simulink model "Dyn_PointMass_R2015B"  (R2015b)
settings: Solver=ode4  SolverMode=SingleTasking  StartTime=0.0  StopTime=simInit.TSIM  FixedStep=simInit.dt  MaxStep=simInit.dt  RelTol=1e-3
InitFcn:
  | close all
undefined symbols (not defined in the file): base_windspeed, constr, DE2019, DiscIntNeverNeededParam, ENVMT, Lbooth, loiterStates, params, simInit, T, winchParameter
libraries: simulink x40, simulink_extras x3, dspsigops x1
(part 3 of 5)

== system Dyn_PointMass_R2015B/AirborneSystem/FlightControlSystem/PathFollowingController_SS_2/FlightOnFlatEarth (Retraction&Loitering)/CalculateAttitudeCmds/FlightPathLoopRetraction_Aerodynamic/FlightPathLoopRetraction ==
  F_t_kite : Inport
  F_t_set : Inport  Port=2
  nu_a_path : Inport  Port=3
  flightMode : Inport  Port=4
  sub_flightMode : Inport  Port=5
  StateEstimation_Bus : Inport  Port=6
  Bus Selector : BusSelector  OutputSignals=pos_G_O_m,pathangles_a,airdata,mu_a
  Chart : Stateflow chart  TreatAsAtomicUnit=on
  Compare To Constant1 : simulink/Logic and Bit Operations/Compare To Constant  relop===  const=7  OutDataTypeStr=boolean
  Compare To Constant2 : simulink/Logic and Bit Operations/Compare To Constant  relop===  const=6  OutDataTypeStr=boolean
  Delay : Delay  DelayLength=1  InitialConditionSource=Input port
      settings: InputPortMap=u0,p4
  Delay1 : Delay  DelayLength=1  InitialConditionSource=Input port
      settings: InputPortMap=u0,p4
  Demux : Demux  Outputs=2
  Demux1 : Demux  Outputs=2
  Logical Operator : Logic  Operator=OR  AllPortsSameDT=off  OutDataTypeStr=boolean
  MATLAB Function : MATLAB Function  TreatAsAtomicUnit=on
  Scope : Scope  NumInputPorts=3
  Scope1 : Scope
  Switch : Switch  Criteria=u2 > Threshold
  Transfer Fcn : TransferFcn  Commented=through  Numerator=[10]  Denominator=[1 10]
  inversionPathDynamics : MATLAB Function  TreatAsAtomicUnit=on
  mu_a_c : Outport  PortDimensions=1
  alpha_a_c : Outport  Port=2  PortDimensions=1
  chi_dot_real : Outport  Port=3  PortDimensions=1
  gamma_dot_real : Outport  Port=4  PortDimensions=1
  wires:
  Bus Selector/1 -> inversionPathDynamics/6(pos_O)  "<pos_G_O_m>"
  Demux1/2 -> inversionPathDynamics/8(gamma_a)
  Bus Selector/2 -> Demux1/1  "<pathangles_a>"
  Bus Selector/3 -> inversionPathDynamics/9(airdata), MATLAB Function/1(airdata)  "<airdata>"
  StateEstimation_Bus/1 -> Bus Selector/1
  MATLAB Function/1(L_rq) -> Delay/2
  inversionPathDynamics/1(mu_a_c) -> Delay1/1, mu_a_c/1
  Delay1/1 -> inversionPathDynamics/1(mu_a_c_old)
  Delay/1 -> inversionPathDynamics/11(Lrq_old)
  flightMode/1 -> inversionPathDynamics/3(flightMode)
  nu_a_path/1 -> Demux/1
  Demux/2 -> inversionPathDynamics/5(nu_gamma_a)
  Demux/1 -> inversionPathDynamics/4(nu_chi_a)
  inversionPathDynamics/2(alpha_a_c) -> alpha_a_c/1
  Demux1/1 -> inversionPathDynamics/7(chi_a)
  Bus Selector/4 -> inversionPathDynamics/10(mu_a), Delay1/2  "<mu_a>"
  inversionPathDynamics/5(L_rq) -> Delay/1
  inversionPathDynamics/3(chi_dot_real) -> chi_dot_real/1
  inversionPathDynamics/4(gamma_dot_real) -> gamma_dot_real/1
  F_t_set/1 -> Scope/1, Chart/1(Ftset)
  F_t_kite/1 -> Switch/1, Chart/2(Ftm)
  Chart/1(fset) -> Switch/3, Scope/2
  Switch/1 -> Scope/3, inversionPathDynamics/2(f_t)
  sub_flightMode/1 -> Scope1/1, Chart/3(sub_flightMode), Compare To Constant1/1, Compare To Constant2/1
  Compare To Constant2/1 -> Logical Operator/2
  Compare To Constant1/1 -> Logical Operator/1
  Logical Operator/1 -> Switch/2

== system Dyn_PointMass_R2015B/AirborneSystem/FlightControlSystem/PathFollowingController_SS_2/FlightOnFlatEarth (Retraction&Loitering)/CalculateAttitudeCmds/FlightPathLoopRetraction_Aerodynamic/FlightpathReferenceModels ==
  chi_cmd : Inport
  gamma_cmd : Inport  Port=2
  gamma_hedge : Inport  Port=3
  chi_hedge : Inport  Port=4
  Mux2 : Mux  Inputs=2
  Mux3 : Mux  Inputs=2
  SecondOrderReferenceModel_course : Subsystem  mask{omega0_max=params.w0_chi_retraction_max, zeta0=1, y_max=inf, y_min=-inf, yd_max=inf, yd_min=-inf, y2d_max=inf, y2d_min=-inf}
  SecondOrderReferenceModel_pathangle : Subsystem  mask{omega0_max=params.w0_gamma_retraction_max, zeta0=1, y_max=inf, y_min=-inf, yd_max=inf, yd_min=-inf, y2d_max=inf, y2d_min=-inf}
  xD_ref : Outport
  x_ref : Outport  Port=2
  wires:
  gamma_hedge/1 -> SecondOrderReferenceModel_pathangle/2(hedge)
  chi_hedge/1 -> SecondOrderReferenceModel_course/2(hedge)
  gamma_cmd/1 -> SecondOrderReferenceModel_pathangle/1(y_cmd)
  chi_cmd/1 -> SecondOrderReferenceModel_course/1(y_cmd)
  Mux3/1 -> xD_ref/1
  Mux2/1 -> x_ref/1
  SecondOrderReferenceModel_course/1(y_ref) -> Mux2/1
  SecondOrderReferenceModel_pathangle/1(y_ref) -> Mux2/2
  SecondOrderReferenceModel_course/2(y_ref_dot) -> Mux3/1
  SecondOrderReferenceModel_pathangle/2(y_ref_dot) -> Mux3/2

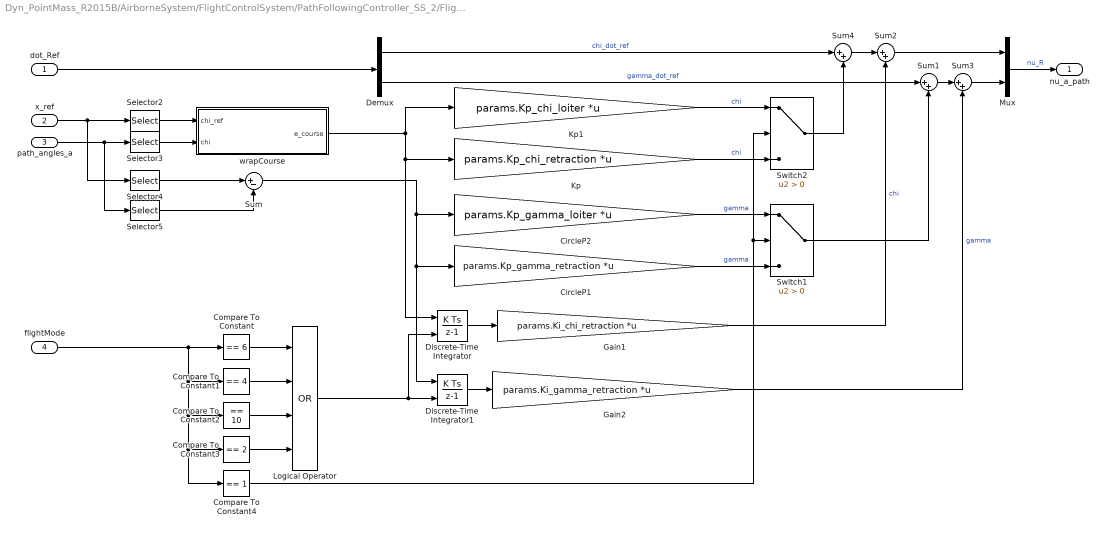
== system Dyn_PointMass_R2015B/AirborneSystem/FlightControlSystem/PathFollowingController_SS_2/FlightOnFlatEarth (Retraction&Loitering)/CalculateAttitudeCmds/FlightPathLoopRetraction_Aerodynamic/PIController_opt ==
  dot_Ref : Inport
  x_ref : Inport  Port=2
  path_angles_a : Inport  Port=3
  flightMode : Inport  Port=4
  CircleP1 : Gain  Gain=params.Kp_gamma_retraction  Multiplication=Matrix(K*u)
  CircleP2 : Gain  Gain=params.Kp_gamma_loiter  Multiplication=Matrix(K*u)
  Compare To Constant : simulink/Logic and Bit Operations/Compare To Constant  relop===  const=6  OutDataTypeStr=boolean
  Compare To Constant1 : simulink/Logic and Bit Operations/Compare To Constant  relop===  const=4  OutDataTypeStr=boolean
  Compare To Constant2 : simulink/Logic and Bit Operations/Compare To Constant  relop===  const=10  OutDataTypeStr=boolean
  Compare To Constant3 : simulink/Logic and Bit Operations/Compare To Constant  relop===  const=2  OutDataTypeStr=boolean
  Compare To Constant4 : simulink/Logic and Bit Operations/Compare To Constant  relop===  const=1  OutDataTypeStr=boolean
  Demux : Demux  Outputs=2
  Discrete-Time Integrator : DiscreteIntegrator  ExternalReset=either  InitialConditionSetting=State (most efficient)  SampleTime=-1  ICPrevOutput=DiscIntNeverNeededParam  ICPrevScaledInput=DiscIntNeverNeededParam
  Discrete-Time Integrator1 : DiscreteIntegrator  ExternalReset=either  InitialConditionSetting=State (most efficient)  SampleTime=-1  ICPrevOutput=DiscIntNeverNeededParam  ICPrevScaledInput=DiscIntNeverNeededParam
  Gain1 : Gain  Gain=params.Ki_chi_retraction  Multiplication=Matrix(K*u) (u vector)
  Gain2 : Gain  Gain=params.Ki_gamma_retraction  Multiplication=Matrix(K*u) (u vector)
  Kp : Gain  Gain=params.Kp_chi_retraction  Multiplication=Matrix(K*u)
  Kp1 : Gain  Gain=params.Kp_chi_loiter  Multiplication=Matrix(K*u)
  Logical Operator : Logic  Operator=OR  Inputs=4  AllPortsSameDT=off  OutDataTypeStr=boolean
  Mux : Mux  Inputs=2
  Selector2 : Selector  InputPortWidth=2  IndexOptions=Index vector (dialog)  Indices=1  OutputSizes=1
  Selector3 : Selector  InputPortWidth=2  IndexOptions=Index vector (dialog)  Indices=1  OutputSizes=1
  Selector4 : Selector  InputPortWidth=2  IndexOptions=Index vector (dialog)  Indices=2  OutputSizes=1
  Selector5 : Selector  InputPortWidth=2  IndexOptions=Index vector (dialog)  Indices=2  OutputSizes=1
  Sum : Sum  Inputs=|+-
  Sum{1..4} (4 alike) : Sum  Inputs=|++
  Switch1 : Switch  Criteria=u2 > Threshold
  Switch2 : Switch  Criteria=u2 > Threshold
  wrapCourse : MATLAB Function  TreatAsAtomicUnit=on
  nu_a_path : Outport
  wires:
  Compare To Constant3/1 -> Logical Operator/4
  Logical Operator/1 -> Discrete-Time Integrator/2, Discrete-Time Integrator1/2
  flightMode/1 -> Compare To Constant2/1, Compare To Constant4/1, Compare To Constant3/1, Compare To Constant1/1, Compare To Constant/1
  Mux/1 -> nu_a_path/1  "nu_R"
  dot_Ref/1 -> Demux/1
  Demux/1 -> Sum4/1  "chi_dot_ref"
  Kp/1 -> Switch2/3  "chi"
  Sum4/1 -> Sum2/1
  wrapCourse/1(e_course) -> Kp/1, Discrete-Time Integrator/1, Kp1/1
  Demux/2 -> Sum1/1  "gamma_dot_ref"
  CircleP1/1 -> Switch1/3  "gamma"
  Sum1/1 -> Sum3/1
  Sum/1 -> Discrete-Time Integrator1/1, CircleP1/1, CircleP2/1
  Compare To Constant/1 -> Logical Operator/1
  Compare To Constant1/1 -> Logical Operator/2
  Compare To Constant2/1 -> Logical Operator/3
  Discrete-Time Integrator1/1 -> Gain2/1
  path_angles_a/1 -> Selector5/1, Selector3/1
  Selector4/1 -> Sum/1
  Selector2/1 -> wrapCourse/1(chi_ref)
  x_ref/1 -> Selector4/1, Selector2/1
  Gain1/1 -> Sum2/2  "chi"
  Gain2/1 -> Sum3/2  "gamma"
  Discrete-Time Integrator/1 -> Gain1/1
  Sum2/1 -> Mux/1
  Sum3/1 -> Mux/2
  Selector5/1 -> Sum/2
  Selector3/1 -> wrapCourse/2(chi)
  Compare To Constant4/1 -> Switch2/2, Switch1/2
  Switch2/1 -> Sum4/2
  Kp1/1 -> Switch2/1  "chi"
  CircleP2/1 -> Switch1/1  "gamma"
  Switch1/1 -> Sum1/2

== system Dyn_PointMass_R2015B/AirborneSystem/FlightControlSystem/PathFollowingController_SS_2/FlightOnFlatEarth (Retraction&Loitering)/GuidanceFlatEarth/LoiteringGuidance/Subsystem ==
  v_k_O : Inport
  h_cmd : Inport  Port=2
  h : Inport  Port=3
  Asin : Trigonometry  Operator=asin
  Divide : Product  Inputs=*/
  Dot Product : DotProduct  InputSameDT=on  OutDataTypeStr=Inherit: Inherit via internal rule
  Gain2 : Gain  Gain=-1
  Gain3 : Gain  Gain=loiterStates.kp_h
  Saturation : Saturate  UpperLimit=50*pi/180  LowerLimit=-50*pi/180
  Saturation1 : Saturate  UpperLimit=1  LowerLimit=-1
  Selector : Selector  InputPortWidth=3  IndexOptions=Index vector (dialog)  Indices=3  OutputSizes=1
  Sqrt : Sqrt  SaturateOnIntegerOverflow=on
  Sum2 : Sum  Inputs=|-+
  gamma_k_cmd : Outport
  wires:
  h_cmd/1 -> Sum2/2
  Saturation/1 -> gamma_k_cmd/1
  Selector/1 -> Gain2/1
  Gain2/1 -> Sum2/1
  Sum2/1 -> Gain3/1
  Sqrt/1 -> Divide/2
  Divide/1 -> Saturation1/1
  Dot Product/1 -> Sqrt/1
  v_k_O/1 -> Dot Product/1, Dot Product/2
  h/1 -> Selector/1
  Asin/1 -> Saturation/1
  Saturation1/1 -> Asin/1
  Gain3/1 -> Divide/1

== system Dyn_PointMass_R2015B/AirborneSystem/FlightControlSystem/PathFollowingController_SS_2/FlightOnFlatEarth (Retraction&Loitering)/GuidanceFlatEarth/Retraction_Nav/Subsystem ==
  In1 : Inport
  Dot Product3 : DotProduct  InputSameDT=on  OutDataTypeStr=Inherit: Inherit via internal rule
  Sqrt1 : Sqrt  SaturateOnIntegerOverflow=on
  Out1 : Outport
  wires:
  In1/1 -> Dot Product3/1, Dot Product3/2
  Sqrt1/1 -> Out1/1
  Dot Product3/1 -> Sqrt1/1

== system Dyn_PointMass_R2015B/AirborneSystem/FlightControlSystem/PathFollowingController_SS_2/FlightOnFlatEarth (Retraction&Loitering)/GuidanceFlatEarth/Retraction_Nav/hold1 ==
  In1 : Inport
  Delay2 : Delay  DelayLength=1  InitialConditionSource=Input port  InitialCondition=zeros(3,1)
      settings: InputPortMap=u0,p4
  Out1 : Outport
  wires:
  In1/1 -> Delay2/2
  Delay2/1 -> Out1/1, Delay2/1

== system Dyn_PointMass_R2015B/AirborneSystem/FlightControlSystem/PathFollowingController_SS_2/FlightOnFlatEarth (Retraction&Loitering)/CalculateAttitudeCmds/FlightPathLoopRetraction_Aerodynamic/FlightpathReferenceModels/SecondOrderReferenceModel_course ==
  y_cmd : Inport
  hedge : Inport  Port=2
  Constant : Constant  Value=omega0_max
  Discrete-Time Integrator : DiscreteIntegrator  InitialConditionSetting=State (most efficient)  SampleTime=-1  LimitOutput=on  UpperSaturationLimit=y_max  LowerSaturationLimit=y_min  ICPrevOutput=DiscIntNeverNeededParam  ICPrevScaledInput=DiscIntNeverNeededParam
  Discrete-Time Integrator1 : DiscreteIntegrator  InitialConditionSetting=State (most efficient)  SampleTime=-1  LimitOutput=on  UpperSaturationLimit=yd_max  LowerSaturationLimit=yd_min  ICPrevOutput=DiscIntNeverNeededParam  ICPrevScaledInput=DiscIntNeverNeededParam
  Gain2 : Gain  Gain=2*zeta0
  Product : Product  Inputs=3
  Product1 : Product
  Saturation : Saturate  UpperLimit=y_max  LowerLimit=y_min
  Saturation1 : Saturate  UpperLimit=y2d_max  LowerLimit=y2d_min
  Sum : Sum  Inputs=|+-
  Sum2 : Sum  Inputs=|+-
  calcualteCourseErrorAndWrap : MATLAB Function  TreatAsAtomicUnit=on
  wrapto2pi : MATLAB Function  TreatAsAtomicUnit=on
  y_ref : Outport
  y_ref_dot : Outport  Port=2
  wires:
  Product1/1 -> Gain2/1
  Constant/1 -> Product1/2, Product/3, Product/1
  Discrete-Time Integrator/1 -> wrapto2pi/1(u)
  Product/1 -> Sum/1
  y_cmd/1 -> Saturation/1
  Discrete-Time Integrator1/1 -> y_ref_dot/1, Product1/1, Sum2/1  "v:_r"
  Sum/1 -> Saturation1/1
  Gain2/1 -> Sum/2
  calcualteCourseErrorAndWrap/1(e_course) -> Product/2
  Saturation1/1 -> Discrete-Time Integrator1/1  "v_dot_r"
  Saturation/1 -> calcualteCourseErrorAndWrap/1(chi_ref)
  Sum2/1 -> Discrete-Time Integrator/1
  hedge/1 -> Sum2/2
  wrapto2pi/1(y) -> calcualteCourseErrorAndWrap/2(chi), y_ref/1

== system Dyn_PointMass_R2015B/AirborneSystem/FlightControlSystem/PathFollowingController_SS_2/FlightOnFlatEarth (Retraction&Loitering)/CalculateAttitudeCmds/FlightPathLoopRetraction_Aerodynamic/FlightpathReferenceModels/SecondOrderReferenceModel_pathangle ==
  y_cmd : Inport
  hedge : Inport  Port=2
  Constant : Constant  Value=omega0_max
  Discrete-Time Integrator : DiscreteIntegrator  InitialConditionSetting=State (most efficient)  SampleTime=-1  LimitOutput=on  UpperSaturationLimit=y_max  LowerSaturationLimit=y_min  ICPrevOutput=DiscIntNeverNeededParam  ICPrevScaledInput=DiscIntNeverNeededParam
  Discrete-Time Integrator1 : DiscreteIntegrator  InitialConditionSetting=State (most efficient)  SampleTime=-1  LimitOutput=on  UpperSaturationLimit=yd_max  LowerSaturationLimit=yd_min  ICPrevOutput=DiscIntNeverNeededParam  ICPrevScaledInput=DiscIntNeverNeededParam
  Gain2 : Gain  Gain=2*zeta0
  Product : Product  Inputs=3
  Product1 : Product
  Saturation : Saturate  UpperLimit=y_max  LowerLimit=y_min
  Saturation1 : Saturate  UpperLimit=y2d_max  LowerLimit=y2d_min
  Sum : Sum  Inputs=|+-
  Sum1 : Sum  Inputs=|+-
  Sum2 : Sum  Inputs=|+-
  y_ref : Outport
  y_ref_dot : Outport  Port=2
  wires:
  Product1/1 -> Gain2/1
  Constant/1 -> Product1/2, Product/3, Product/1
  Product/1 -> Sum/1
  y_cmd/1 -> Saturation/1
  Discrete-Time Integrator1/1 -> y_ref_dot/1, Product1/1, Sum2/1  "v:_r"
  Sum/1 -> Saturation1/1
  Gain2/1 -> Sum/2
  Sum1/1 -> Product/2
  Saturation1/1 -> Discrete-Time Integrator1/1  "v_dot_r"
  Saturation/1 -> Sum1/1
  Sum2/1 -> Discrete-Time Integrator/1
  hedge/1 -> Sum2/2
  Discrete-Time Integrator/1 -> y_ref/1, Sum1/2

== stateflow chart Dyn_PointMass_R2015B/AirborneSystem/FlightControlSystem/PathFollowingController_SS_2/FlightOnFlatEarth (Retraction&Loitering)/CalculateAttitudeCmds/FlightPathLoopRetraction_Aerodynamic/FlightPathLoopRetraction/Chart ==
  settings: updateMethod=DISCRETE  sampleTime=0.1
  state ReducedSetforce
    during: fset = 0 ;
    during: t = t + 1;
  state Setforce
    during: fset = Ftset;
    entry: t=0;
  Setforce -> ReducedSetforce [commented out] : [Ftm>Ftset+1000]
  (default) -> Setforce
  Setforce -> ReducedSetforce : [sub_flightMode==6 || sub_flightMode == 7]
  ReducedSetforce -> Setforce : [sub_flightMode==8]
  ReducedSetforce -> Setforce [commented out] : [Ftm<Ftset-1000]
  data: Ftset input; Ftm input; fset output; t local; sub_flightMode input

== matlab function Dyn_PointMass_R2015B/ParticleTetherModel/Tether_SS_5/Tether_Dynamics ==
  data: kitePos input; tetherPos output size=[3,T.np]; kiteVel input; windVel input; tetherLength input; x input; Ft_Ground output; Ft_Kite output; Fvec output; x output; ENVMT parameter; T parameter
% Copyright 2021 Delft University of Technology
%
% Licensed under the Apache License, Version 2.0 (the "License");
% you may not use this file except in compliance with the License.
% You may obtain a copy of the License at
%
%      http://www.apache.org/licenses/LICENSE-2.0
%
% Unless required by applicable law or agreed to in writing, software
% distributed under the License is distributed on an "AS IS" BASIS,
% WITHOUT WARRANTIES OR CONDITIONS OF ANY KIND, either express or implied.
% See the License for the specific language governing permissions and
% limitations under the License.

function [tetherPos, Ft_Ground, Ft_Kite, Fvec, x]= ...
    Tether_QuasiStatic(kitePos, kiteVel, windVel, tetherLength, x, ENVMT, T)
%#codegen

%Tether_QuasiStatic Trust-region dogleg nonlinear systems of equation
%   solver to determine the tether shape and forces.
%
%   Tether_QuasiStatic is based on the matlab implementation that 
%   solves a system of nonlinear equations using a dogleg
%   trust region approach.  The algorithm implemented is similar in nature
%   to the FORTRAN program HYBRD1 of J.J. More', B.S. Garbow and K.E. 
%   Hillstrom, User Guide for MINPACK 1, Argonne National Laboratory, 
%   Rept. ANL-80-74, 1980, which itself was based on the program CALFUN 
%   of M.J.D. Powell, A Fortran subroutine for solving systems of
%   nonlinear algebraic equations, Chap. 7 in P. Rabinowitz, ed.,
%   Numerical Methods for Nonlinear Algebraic Equations, Gordon and
%   Breach, New York, 1970.
%
%   Addapted by Ir. D. Eijkelhof (TU Delft) from 1990-2019 Matlab version 
%   The MathWorks, Inc.
% NOTE: From Matlab 2020b Matlab's Levenberg–Marquardt algorithm in the
% command "solve" can be directly used in codegen and might be
% faster. Due to availability of only matlab R2019B and lower, an own
% implementation had to be used in order the execute codegen.
%
% Syntax:  [tetherPos, Ft_Ground, Ft_Kite, Fvec, x]= ...
%     Tether_QuasiStatic(kitePos, kiteVel, windVel, tetherLength, x, ENVMT, T)
%
% NOTE: 'x' passed in and returned in column vector form.
%
% Throughout this routine 'x', 'F', 'xvec', 'xTrial', 'Fvec' and 'FTrial' are vectors.
%
% Inputs:
%    tetherPos  - Position vectors of tether particles
%    Ft_Ground  - Tether force magnitude at the ground station
%    Ft_Kite    - Tether force vector at the kite
%    Fvec       - Error between tether end and kite position (3D)
%    x          - Tether ground segment orientation and magnitude
%
% Outputs:
%    kitePos        - Kite position vector in wind reference frame
%    kiteVel        - Kite velocity vector in wind reference frame
%    windVel        - Wind velocity vector in wind reference frame
%    ENVMT          - Environmental parameters
%    tetherLength   - Reeled-out tether length determined by the winch
%    x              - Initial tether ground segment orientation and magnitude
%    T              - Tether dimensions and material properties
%
% Other m-files required: none
%
% Subfunctions: Objfunc    : Calculate difference between tether end and
%                            kite given tether ground segment orientation
%                            and magnitude.
%               testStop   : Test convergence criteria's
%               dogleg_tem : approximately solves trust region subproblem
%                            via a dogleg approach. 
%               lm_FD_J    : Determines the jacobian matrix by forward
%                            differencing
%
% MAT-files required: none
%
% Author: Dylan Eijkelhof, M.Sc.
% Delft University of Technology
% email address: d.eijkelhof@tudelft.nl  
% December 2019; Last revision: 16-March-2021

%------------- BEGIN CODE --------------
    
    [Fvec,T0,pj,~] = Objfunc(x,kitePos,kiteVel,windVel,tetherLength,ENVMT,T);
    
    xvec = x(:);         % vector representation of x
    % Convert values to full to avoid unnecessary sparse operation overhead
    % Initial x
    Fvec = full(Fvec); 
    
    % Set tolerances
    maxfunc     = 100*5;
    maxit       = 1000;
    tolf        = 1e-9;
    tolfunvalue = 1e-6;
    tolx        = 1e-6;
    tolobj      = 1e-6;
    
    nVar        = 3; % for codegen it worked better than numel(x)

    % Initialize local arrays.
    d           = zeros(nVar,1);

    % Initialize other trust region parameters.
    Delta       = 1e0;
    DeltaMax    = 1e10;
    eta1        = T.eta1;
    eta2        = T.eta2;
    alpha1      = T.alpha1;
    alpha2      = T.alpha2;

    % Extra initializations.
    iter        = 0;
    numFevals   = 1;

    stepAccept  = true;
    normd       = 0.0e0;
    objold      = 1.0e0;
    obj         = 0.5*(Fvec'*Fvec);  % Initial Fvec computed above

    numFDfevals = 0; %#ok<NASGU>
    JAC         = zeros(3,3); %#ok<PREALL> % pre-allocate derivative array

    %%%%%%%%%%%%%%%%%%%%%%% Calculate Jacobian at x0 %%%%%%%%%%%%%%%%%%
    [JAC,numFDfevals] = lm_FD_J(x, 0.1*ones(3,1),kitePos, kiteVel, ...
        windVel, tetherLength, ENVMT, T);

    % Increment the number of function evaluations with those used in the
    % finite difference calls.
    numFevals = numFevals + numFDfevals;

    grad = JAC'*Fvec;
    normgradinf = norm(grad,inf);

    % Test convergence at initial point.
    [done,~] = testStop(normgradinf,tolf,tolfunvalue,tolx,...
         stepAccept,iter,maxit,numFevals,maxfunc,Delta,normd,...
         obj,objold,d,xvec,tolobj,Fvec);

    % Beginning of main iteration loop.
    while ~done
    	iter = iter + 1;

    	% Compute step, d, using dogleg approach.
    	[d,quadObj,normd,normdscal] = ...
           dogleg(nVar,Fvec,JAC,grad,Delta);

        % Compute the model reduction given by d (pred).
        pred = -quadObj;

        % Compute the trial point, xTrial. Limit to positive value
        xTrial = xvec + d;
        if xTrial(3) < 0
            xTrial(3) = 1e-3;
        end

        % Evaluate nonlinear equations and objective at trial point.
        [F,T0,pj,~] = Objfunc(xTrial,kitePos,kiteVel,windVel,tetherLength,...
            ENVMT,T);
      
      
        numFevals = numFevals + 1;
        FTrial    = full(F(:)); % make FTrial a vector, convert to full
        objTrial  = 0.5*(FTrial'*FTrial); 

        % Compute the actual reduction given by xTrial (ared).
        ared      = obj - objTrial;

        % Compute ratio = ared/pred.
        if pred <= 0 % reject step
            ratio = 0;
        else
            ratio = ared/pred;
        end

        currTrialWellDefined = isfinite(objTrial);

        if ratio > eta1 && currTrialWellDefined % accept step.

            xvec    = xTrial; 
            objold  = obj; 
            obj     = objTrial;
            x(:)    = xvec; % update matrix representation
        
            %%%%%%%%%%%%%%%%%%%%%% Calculate New Jacobian %%%%%%%%%%%%%%%%%
            if iter == 1 || mod(iter,2*size(x,1))==0
                [JAC,numFDfevals] = lm_FD_J(x, 0.01*ones(3,1),kitePos, kiteVel, windVel, tetherLength, ENVMT, T);

                numFevals = numFevals + numFDfevals;
            else
                JAC = JAC + ((FTrial-Fvec-JAC*d)*d')/(d'*d);
            end
        
            Fvec        = FTrial; 
            grad        = JAC'*Fvec;
            normgradinf = norm(grad,inf);

            stepAccept  = true;
        else % reject step.
            stepAccept  = false;
        end 


        % Update trust region radius.
        if ~currTrialWellDefined
            % Shrink the trust region if any element of the function vector
            % at the new step is not defined (i.e. it's inf/NaN/complex). The
            % update for Delta in this case follows that in snls.
            Delta = min(normdscal/20,Delta/20);
        elseif ratio < eta1
            Delta = alpha2*normdscal;
        elseif ratio >= eta2
            Delta = max(Delta,alpha1*normdscal);
        end
        Delta = min(Delta,DeltaMax);

        % Check for termination.
        [done,~] = testStop(normgradinf,tolf,tolfunvalue,tolx,...
            stepAccept,iter,maxit,numFevals,maxfunc,Delta,normd,...
            obj,objold,d,xvec,tolobj,Fvec);
    end

    % Optimization is finished.  
    Ft_Ground   = x(3);
    Ft_Kite     = T0;
    tetherPos   = pj;
end

%%%%%%%%%%%%%%%%%%%%%%%%%%%%%%%%%%%%%%%%%%%%%%%%%%%%%%%%%%%%%%%
function [Fobj,T0,pj,p0] = Objfunc(stateVec,kitePos, kiteVel, windVel,...
                              tetherLength, ENVMT, T)
    Ns = size(windVel,2);       % number of masses
    Ls = tetherLength/(Ns+1);   % segment length
    mj = T.rho_t * Ls;          % segment mass

    p = kitePos;                % input aircraft position
    v = kiteVel;                % input aircraft velocity

    theta = stateVec(1);
    phi = stateVec(2);
    Tn = stateVec(3);

    omega_t = cross(p./(norm(p)^2),v);

    E = T.E;
    A = T.A;

    FT = zeros(3,Ns); % Tension forces
    Fd = zeros(3,Ns); % Drag forces
    pj = zeros(3,Ns); % Mass positions
    vj = zeros(3,Ns); % Mass velocities
    aj = zeros(3,Ns); % Mass accellerations

    % First element from ground station (Ns)
    FT(:,Ns) = Tn.*[sin(theta)* cos(phi); sin(phi); cos(theta)*cos(phi)];
    pj(:,Ns) = Ls.*[sin(theta)* cos(phi); sin(phi); cos(theta)*cos(phi)];
    vj(:,Ns) = dot(v,p./norm(p)) .* (p./norm(p)) + cross(omega_t,pj(:,Ns));
    aj(:,Ns) = cross(omega_t,cross(omega_t,pj(:,Ns)));
    
    % Drag calculation first element
    v_a_p = vj(:,Ns) - windVel(:,Ns);
    if all(abs(v_a_p)<1e-3)
        Fd(:,Ns) = [0;0;0];
    else
        v_a_p_t = dot((pj(:,Ns))/norm(pj(:,Ns)),v_a_p)*...
            ((pj(:,Ns))/norm(pj(:,Ns)));
        v_a_p_n = v_a_p - v_a_p_t;
        Fd(:,Ns) = -0.5 * ENVMT.rhos * Ls * T.d_tether * T.CD_tether * ...
            norm(v_a_p_n) * v_a_p_n; % particle drag
    end
    
    % All other segments and masses except for segment connected to the kite
    for i = Ns:-1:2
        if i == Ns
            FT(:,i-1) = (mj+0.5*mj).*aj(:,i) + FT(:,i) - Fd(:,i) + ...
                [0;0;(mj+0.5*mj)*ENVMT.g];
        else
            FT(:,i-1) = mj.*aj(:,i) + FT(:,i) - Fd(:,i) + [0;0;mj*ENVMT.g];
        end

        l_i_1 = (norm(FT(:,i-1))/(E*A) + 1)*Ls;
        
        pj(:,i-1) = pj(:,i) + l_i_1.*(FT(:,i-1)/norm(FT(:,i-1)));       
        vj(:,i-1) = dot(v,p./norm(p)) .* (p./norm(p)) + cross(omega_t,pj(:,i-1));
        aj(:,i-1) = cross(omega_t,cross(omega_t,pj(:,i-1)));
        
        % Drag calculation
        v_a_p = vj(:,i) - windVel(:,i);
        if all(abs(v_a_p)<1e-3)
            Fd(:,i-1) = [0;0;0];
        else
            v_a_p_t = dot((pj(:,i-1)-pj(:,i))/norm(pj(:,i-1)-pj(:,i)),v_a_p) * ...
                ((pj(:,i-1)-pj(:,i))/norm(pj(:,i-1)-pj(:,i)));
            v_a_p_n = v_a_p - v_a_p_t;
            Fd(:,i-1) = -0.5 * ENVMT.rhos * Ls * T.d_tether * T.CD_tether * ...
                norm(v_a_p_n) * v_a_p_n; % particle drag
        end
    end
    
    T0 = (mj+0.5*mj).*aj(:,1) + FT(:,1) - Fd(:,1) + [0;0;(mj+0.5*mj)*ENVMT.g];
    l_i_1 = (norm(T0)/(E*A) + 1)*Ls;
    p0 = pj(:,1) + l_i_1.*(T0/norm(T0));
    
    Fobj = p-p0;
end
%%%%%%%%%%%%%%%%%%%%%%%%%%%%%%%%%%%%%%%%%%%%%%%%%%%%%%%%%%%%%%%
function [done,EXITFLAG] = testStop(normgradinf,tolf,tolfunvalue,...
        tolx,stepAccept,iter,maxit,numFevals,maxfunc,Delta,normd,...
        obj,objold,d,xvec,tolobj,Fvec)
    %testStop checks the termination criteria for TRUSTNLEQN.

    done = false;
    EXITFLAG = 0;

    % Check termination criteria.

    if stepAccept && normgradinf < tolf
      EXITFLAG = 1;
      done = true;
      
    elseif iter > 1 && max(abs(d)./(abs(xvec)+1)) < max(tolx^2,eps)
       EXITFLAG = 2;
       done = true;
       
    elseif iter > 1 && stepAccept && normd < 0.9*Delta ...
                    && abs(objold-obj) < max(tolfunvalue^2,eps)*(1+abs(objold))
      EXITFLAG = 3;
      done = true;
      
    elseif iter > 1 && norm(Fvec) < tolobj
      EXITFLAG = 4;
      done = true;
      
    elseif Delta < 2*eps
      EXITFLAG = -3;
      done = true;
      
    elseif iter >= maxit
      EXITFLAG = 0;
      done = true;
      
    elseif numFevals >= maxfunc
      EXITFLAG = 0;
      done = true;
    end  
end
%%%%%%%%%%%%%%%%%%%%%%%%%%%%%%%%%%%%%%%%%%%%%%%%%%%%%%%%%%%%%%%
function [step,quadObj,normStep,normStepScal] = ...
    dogleg(nvar,F,JAC,grad,Delta)
%dogleg approximately solves trust region subproblem via a dogleg approach.
%
%   dogleg finds an approximate solution d to the problem:
%
%     min_d      f + g'd + 0.5*d'Bd
%
%     subject to ||Dd|| <= Delta
%
%   where g is the gradient of f, B is a Hessian approximation of f, D is a
%   diagonal scaling matrix and Delta is a given trust region radius.

%   Copyright 1990-2012 The MathWorks, Inc.
%   $Revision: 1.1.6.7 $  $Date: 2012/08/21 01:08:20 $

% NOTE: The scaling matrix D above is called scalMat in this routine.

% Compute scaled gradient and other scaled terms.
grad2 = grad;
normgradscal = norm(grad);

if normgradscal >= eps
    % First compute the Cauchy step (in scaled space).
    dCauchy = -(Delta/normgradscal)*grad;
    JACvec = JAC*grad2;
    denom = Delta*(JACvec'*JACvec);
    tauterm = normgradscal^3/denom;
    tauC = min(1,tauterm);
    dCauchy = tauC*dCauchy;
    
    % Compute quadratic objective at Cauchy point.
    JACvec = JAC*(dCauchy); 
    objCauchy = grad'*dCauchy + 0.5*(JACvec'*JACvec);   
    normdCauchy = min(norm(dCauchy),Delta);
else
    % Set Cauchy step to zero step and continue.
    objCauchy = 0;
    normdCauchy = 0;
    dCauchy = zeros(nvar,1);
end

if Delta - normdCauchy < eps
    % Take the Cauchy step if it is at the boundary of the trust region.
    step = dCauchy; quadObj = objCauchy;
else
    % Compute the Gauss-Newton step (in scaled space).
    
    dNewton = -JAC\F;
    
    if any(~isfinite(dNewton))
        % Take the Cauchy step if the Gauss-Newton step gives bad values.
        step = dCauchy; quadObj = objCauchy;
    else 
        normdNewt = norm(dNewton);
        if normdNewt <= Delta
            % Use the Newton direction as the trial step
            step = dNewton;
        else
            % Find the intersect point along dogleg path.
            Delta2 = Delta^2;
            normdCauchy2 = min(normdCauchy^2,Delta2);
            normdNewt2 = normdNewt^2;
            dCdN = dCauchy'*dNewton;
            dCdNdist2 = max((normdCauchy2+normdNewt2-2*dCdN),0);
            
            if dCdNdist2 == 0
                Lambda = 0;
            else
                % Stable method for solving 1-D quadratic
                a = 0.5*dCdNdist2;
                b = dCdN - normdCauchy2;
                c = 0.5*(normdCauchy2 - Delta2);
                q = -0.5*(b + sign(b)*sqrt(b^2 - 4*a*c));
                if b > 0
                    Lambda = c/q; 
                else
                    Lambda = q/a;
                end

                % Make sure we take a finite step,
                % (check for poorly scaled/infinite directions).
                if ~isfinite(Lambda)
                    Lambda = 0; % Take Cauchy step
                end
            end
            step = dCauchy + Lambda*(dNewton-dCauchy);
        end
        % Compute quadratic objective at trial point.
        JACvec = JAC*(step);
        quadObj = grad'*step + 0.5*(JACvec'*JACvec);
        
        % Compare Cauchy step and trial step (Newton or intersection)
        if objCauchy < quadObj
            step = dCauchy; quadObj = objCauchy;
        end
    end
end

% The step computed was the scaled step.  Unscale it.
normStepScal = norm(step);
normStep = norm(step);
end
 %%%%%%%%%%%%%%%%%%%%%%%%%%%%%%%%%%%%%%%%%%%%%%%%%%%%%%%%%%%%%%%
function [J,numFDfevals] = lm_FD_J(x, dp,kitePos, kiteVel, windVel, ...
                                tetherLength, ENVMT, T)

 m      = 3;                         % number of data points
 n      = 3;                         % number of parameters

 ps     = x; 
 J      = zeros(m,n); 
 del    = zeros(n,1);                % initialize Jacobian to Zero
 
 for j=1:n                           % START --- loop over all parameters

   del(j) = dp(j) * (1+abs(x(j)));   % parameter perturbation
   x(j)   = ps(j) + del(j);          % perturb parameter x(j)

   if del(j) ~= 0
     [y1,~,~,~] = Objfunc(x,kitePos, kiteVel, windVel, ...
         tetherLength, ENVMT, T);
     
     x(j) = ps(j) - del(j);
     [y,~,~,~] = Objfunc(x,kitePos, kiteVel, windVel, ...
         tetherLength, ENVMT, T);
     
     J(:,j) = (y1-y) ./ (2 .* del(j));
   end

   x(j) = ps(j);                     % restore x(j)

 end
 numFDfevals = 2;
                                     % END --- loop over all parameters
end

== matlab function Dyn_PointMass_R2015B/AirborneSystem/FlightControlSystem/PathFollowingController_SS_2/FlightOnFlatEarth (Retraction&Loitering)/CalculateAttitudeCmds/FlightPathLoopRetraction_Aerodynamic/FlightPathLoopRetraction/MATLAB Function ==
  data: L_rq output; airdata input; DE2019 parameter; constr parameter; ENVMT parameter
% Copyright 2021 Delft University of Technology
%
% Licensed under the Apache License, Version 2.0 (the "License");
% you may not use this file except in compliance with the License.
% You may obtain a copy of the License at
%
%      http://www.apache.org/licenses/LICENSE-2.0
%
% Unless required by applicable law or agreed to in writing, software
% distributed under the License is distributed on an "AS IS" BASIS,
% WITHOUT WARRANTIES OR CONDITIONS OF ANY KIND, either express or implied.
% See the License for the specific language governing permissions and
% limitations under the License.

function L_rq = fcn(airdata, DE2019,constr, ENVMT)
%fcn - Calculate required lift force
%
% Inputs:
%    airdata     - Airspeed, aoa, sideslip angle
%    DE2019     - Aircraft characteristics
%    constr     - Constraint, maximum lift
%
% Outputs:
%    L_rq    - Required lift
%
% Author: Sebastian Rapp, Ph.D., Revised by: Dylan Eijkelhof, M.Sc.
% Delft University of Technology
% email address: s.rapp@tudelft.nl
% email address: d.eijkelhof@tudelft.nl
% December 2019; Last revision: 06-October-2020

%-------------	BEGIN CODE	--------------

L_rq =  min( 0.5*ENVMT.rhos*DE2019.S_wing*airdata(1)^2 * (DE2019.CL0+DE2019.CL_alpha*airdata(2) ),constr.F_T_max); % max. negative lift

%-------------	 END CODE	--------------
end

== matlab function Dyn_PointMass_R2015B/AirborneSystem/FlightControlSystem/PathFollowingController_SS_2/FlightOnFlatEarth (Retraction&Loitering)/CalculateAttitudeCmds/FlightPathLoopRetraction_Aerodynamic/FlightPathLoopRetraction/inversionPathDynamics ==
  data: mu_a_c_old input; f_t input; flightMode input; nu_chi_a input; mu_a_c output; nu_gamma_a input; DE2019 parameter; pos_O input; chi_a input; gamma_a input; airdata input; mu_a input; constr parameter; alpha_a_c output; chi_dot_real output; gamma_dot_real output; ENVMT parameter; L_rq output; Lrq_old input
% Copyright 2021 Delft University of Technology
%
% Licensed under the Apache License, Version 2.0 (the "License");
% you may not use this file except in compliance with the License.
% You may obtain a copy of the License at
%
%      http://www.apache.org/licenses/LICENSE-2.0
%
% Unless required by applicable law or agreed to in writing, software
% distributed under the License is distributed on an "AS IS" BASIS,
% WITHOUT WARRANTIES OR CONDITIONS OF ANY KIND, either express or implied.
% See the License for the specific language governing permissions and
% limitations under the License.

function [mu_a_c,alpha_a_c,chi_dot_real,gamma_dot_real, L_rq] = ...
    InversePathDynamics(mu_a_c_old, f_t, flightMode,nu_chi_a, nu_gamma_a,DE2019, ...
    pos_O, chi_a, gamma_a, airdata, mu_a, constr,ENVMT, Lrq_old)
%InversePathDynamics - Calculated desired roll and pitch angles 
%
% Inputs:
%    mu_a_c_old  - Old desired aerodynamic roll angle
%    f_t         - Corrected tether force set point
%    flightMode  - Flightmode, 6 during retraction
%    nu_chi_a    - Course angle error
%    nu_gamma_a  - Path angle error
%    DE2019      - Aircraft characteristics
%    pos_O       - Aircraft position in inertial reference frame
%    chi_a       - Course angle
%    gamma_a     - Path angle
%    airdata     - Airspeed, aoa and sideslip angle
%    mu_a        - Current roll angle
%    constr      - Dynamic constraints
%    ENVMT       - Environment characteristics
%    L_rq_old    - Old required lift
%
% Outputs:
%    mu_a_c         - Desired roll angle
%    alpha_a_c      - Desired pitch angle
%    chi_dot_real   - Course angle rate of change
%    gamma_dot_real - Path angle rate of change
%    L_rq           - Required lift
%
% Author: Sebastian Rapp, Ph.D., Revised by: Dylan Eijkelhof, M.Sc.
% Delft University of Technology
% email address: s.rapp@tudelft.nl
% email address: d.eijkelhof@tudelft.nl
% December 2019; Last revision: 06-October-2020

%-------------	BEGIN CODE	--------------
%% Initialise parameters for codegen
chi_dot_real = 0;
gamma_dot_real = 0;
push_mode = 0;
mu_a_c = 0;
L_rq = 0;
alpha_a_c = 0;
ddt_v_w_x_O = 0;

%%
c_chi_a = cos(chi_a); 
c_gamma_a = cos(gamma_a); 
s_chi_a = sin(chi_a); 
s_gamma_a = sin(gamma_a); 

Va = airdata(1); 
alpha = airdata(2);

M_AbarO = [ c_chi_a*c_gamma_a, s_chi_a*c_gamma_a, -s_gamma_a; 
    -s_chi_a, c_chi_a, 0; 
    c_chi_a*s_gamma_a, s_chi_a*s_gamma_a, c_gamma_a];

F_g_Abar = M_AbarO * [0;0;DE2019.mass*ENVMT.g];
F_t_Abar = -M_AbarO * pos_O/norm(pos_O)*f_t; 


fy  =  DE2019.mass * ( nu_chi_a * cos(gamma_a) * Va - sin(chi_a)*ddt_v_w_x_O) - F_g_Abar(2) - F_t_Abar(2)  ;
fz =   DE2019.mass  * (nu_gamma_a * Va              - cos(chi_a)*sin(gamma_a)*ddt_v_w_x_O ) + F_g_Abar(3) + F_t_Abar(3);
mu_a_c = atan2(fy,fz);

push_mode = 0;
L_min =  0.5*ENVMT.rhos*DE2019.S_wing*airdata(1)^2 * (DE2019.CL0+DE2019.CL_alpha*constr.alpha_a_min); % max. negative lift

% Recalculation of fy, 
% fy = fz * tan(mu_a); % delay in pull-up
fy = fz * tan(mu_a_c); % leads to pitch then bank behavior.

F_req = min( sqrt( fy^2 + fz^2 ), constr.max_lift );

if abs(mu_a_c)>constr.mu_a_max_retraction && abs(F_req)<abs(L_min) || (fz < 0 && flightMode == 6) % in the retraction phase we want to burn tether force hence it makes sense to fly in push mode.
    mu_a_tmp = mu_a_c + pi; 
    if mu_a_tmp > pi
        du = mod(mu_a_tmp,pi);
        mu_a_tmp = -pi+du;
    elseif mu_a_tmp < -pi
        du = mod(mu_a_tmp,-pi);
        mu_a_tmp = pi+du;
    end
    if abs(mu_a_tmp) <= constr.mu_a_max_retraction || flightMode == 6
        mu_a_c = mu_a_tmp;
        push_mode = 1;
    end
end

mu_a_c = max( min( mu_a_c , constr.mu_a_max_retraction), -constr.mu_a_max_retraction);

%fy = fz * max( min( tan(mu_a_c), 1), -1); % first pull up then bank
fy = fz * tan(mu_a_c);

F_req = min( sqrt( fy^2 + fz^2 ), constr.max_lift );

if push_mode
    L_rq = -F_req;
else
    L_rq = F_req;
end

% hold old bank angle if required lift is very small, avoid agressive
% banking for small absolute values of L i.e. for small values inaccuracies
% like numerical inaccuracies have a large impact on the mu_a_c.
if abs(L_rq) <= 1
    mu_a_c = mu_a_c_old;
end

% for large bank angle changes only adapt the lift if close to the current
% lift. The lontitudional dynamic is faster, hence if we command large bank
% angles this would result in a large lift which would first create a large
% curvature in the longi plane before the actual curvature in the lateral
% plan is achieved.
if abs( mu_a_c - mu_a ) > constr.max_delta_mu
    L_rq = Lrq_old;
end

CL_rq = max( min( 2*L_rq / ( ENVMT.rhos*DE2019.S_wing*airdata(1)^2 ), constr.max_CL), constr.min_CL);
alpha_a_c = max( min( (CL_rq-DE2019.CL0)/DE2019.CL_alpha, constr.alpha_a_max), constr.alpha_a_min); 
CL = max( min( DE2019.CL0+DE2019.CL_alpha*alpha_a_c, constr.max_CL), constr.min_CL);

Lreal = 0.5 * Va^2 * 1.225 * DE2019.S_wing * CL; 
chi_dot_real = 1/cos(gamma_a)/Va/DE2019.mass*(sin(mu_a_c)*Lreal + F_g_Abar(2) + F_t_Abar(2));
gamma_dot_real = -1/Va/DE2019.mass*(-cos(mu_a_c)*Lreal + F_g_Abar(3) + F_t_Abar(3));

%-------------	 END CODE	--------------
end

== stateflow chart Dyn_PointMass_R2015B/GroundSystem_SS_4/GroundControl/Chart ==
  note: Counter structure that counts the figures of 8
      | during the traction phase and resets as soon as
      | the retraction phase is triggered
  state counter1
    entry: c=c+1;
    entry: c_out = c;
  state counter2
    entry: c=c+1;
    entry: c_out = c;
  state s1
  state init
    entry:c=-1;
    entry: c_out = c;
  state reset
    entry: c=-1;
    entry: c_out = c;
  state counter3
    entry: c=c+1;
    entry: c_out = c;
  state s4
  state counter
    entry: c=c+1;
    entry: c_out = c;
  reset -> s1 [order 1] : [long>0]
  counter1 -> reset [order 1] : [fm==6]
  counter1 -> counter2 [order 2] : [long<0]
  counter2 -> counter1 [order 1] : [long>0]
  s1 -> counter2 : [long<0]
  init -> s1 [order 1] : [long>0]
  counter2 -> reset [order 2] : [fm==6]
  (default) -> init
  reset -> s4 [order 2] : [long<=0]
  counter3 -> reset [order 1] : [fm==6]
  counter -> reset [order 2] : [fm==6]
  init -> s4 [order 2] : [long<=0]
  s4 -> counter3 : [long>0]
  counter -> counter3 [order 1] : [long>0]
  counter3 -> counter [order 2] : [long<0]
  data: long input; fm input; c_out output; c local

== matlab function Dyn_PointMass_R2015B/Environment_SS_3/MATLAB Function ==
  data: vec_W output; vec_O input; wind_direction_rad input
% Copyright 2021 Delft University of Technology
%
% Licensed under the Apache License, Version 2.0 (the "License");
% you may not use this file except in compliance with the License.
% You may obtain a copy of the License at
%
%      http://www.apache.org/licenses/LICENSE-2.0
%
% Unless required by applicable law or agreed to in writing, software
% distributed under the License is distributed on an "AS IS" BASIS,
% WITHOUT WARRANTIES OR CONDITIONS OF ANY KIND, either express or implied.
% See the License for the specific language governing permissions and
% limitations under the License.

function vec_W = transformO2W(vec_O, wind_direction_rad)
%transformO2W - transform inertial reference frame to wind reference frame
%
% Syntax:  vec_W = transformO2W(vec_O, wind_direction_rad)
%
% Inputs:
%    vec_O - Aircraft position in inertial reference frame
%    wind_direction_rad - Wind direction angle compared to intertial
%                         reference frame
%
% Outputs:
%    vec_W  - Propulsive forces in body reference frame
%   
% Example: 
%    vec_W = transformO2W(vec_O, wind_direction_rad)
%
% Other m-files required: none
% Subfunctions: none
% MAT-files required: none
%
% Author: Dylan Eijkelhof, M.Sc.
% Delft University of Technology
% email address: d.eijkelhof@tudelft.nl  
% December 2019; Last revision: 30-September-2019

%------------- BEGIN CODE --------------    

M_WO = [cos(wind_direction_rad), sin(wind_direction_rad), 0;
        sin(wind_direction_rad), -cos(wind_direction_rad), 0;
        0, 0, -1];

vec_W = M_WO*vec_O;
%------------- END CODE --------------   
end

== matlab function Dyn_PointMass_R2015B/AirborneSystem/FlightControlSystem/PathFollowingController_SS_2/FlightOnFlatEarth (Retraction&Loitering)/CalculateAttitudeCmds/FlightPathLoopRetraction_Aerodynamic/FlightpathReferenceModels/SecondOrderReferenceModel_course/calcualteCourseErrorAndWrap ==
  data: chi_ref input; e_course output; chi input
% Copyright 2021 Delft University of Technology
%
% Licensed under the Apache License, Version 2.0 (the "License");
% you may not use this file except in compliance with the License.
% You may obtain a copy of the License at
%
%      http://www.apache.org/licenses/LICENSE-2.0
%
% Unless required by applicable law or agreed to in writing, software
% distributed under the License is distributed on an "AS IS" BASIS,
% WITHOUT WARRANTIES OR CONDITIONS OF ANY KIND, either express or implied.
% See the License for the specific language governing permissions and
% limitations under the License.

function e_course = course_error(chi_ref, chi)
%course_error - Calculate the error between commanded and actual course angle
%
% Inputs:
%    chi_ref  - Required chi
%    chi      - Actual chi
%
% Outputs:
%    e_course - Course (heading) error
%
% Author: Sebastian Rapp, Ph.D., Revised by: Dylan Eijkelhof, M.Sc.
% Delft University of Technology
% email address: s.rapp@tudelft.nl
% email address: d.eijkelhof@tudelft.nl
% December 2019; Last revision: 06-October-2020

%-------------	BEGIN CODE	--------------
%#codegen
% The vectors are lying in the tangential plane attached to the current
% position on the small earth.
p_bearing_vec =   [cos(chi);         sin(chi);         0];
p_bearing_vec = p_bearing_vec/norm(p_bearing_vec); 
ref_bearing_vec = [cos(chi_ref); sin(chi_ref); 0];
ref_bearing_vec = ref_bearing_vec/norm(ref_bearing_vec); 

e_z = cross( ref_bearing_vec, p_bearing_vec ); 

dot_product = dot( ref_bearing_vec, p_bearing_vec ); 
if dot_product > 1 
    dot_product = 1; 
end
if dot_product < -1 
    dot_product = -1; 
end

e_course = - sign( e_z(3) ) * acos( dot_product );
%-------------	 END CODE	--------------
end

== matlab function Dyn_PointMass_R2015B/AirborneSystem/PointMassEOM/PointMassDynamics/PointMassEOM ==
  data: Va input; alpha input; beta input; v_a_dot output; M_OB output; v_k_W output; pos_O output; pos_W output; v_k_B output; chi_k output; gamma_k output; eta_EULER output; v_k_O output; v_w_O input; mu_a input; F_a_B input; F_p_B input; F_t_W input; chi_a input; gamma_a input; long input; lat input; h_tau input; DE2019 parameter; ENVMT parameter; chi_a_dot output; gamma_a_dot output; long_dot output; lat_dot output; h_tau_dot output
% Copyright 2020 Delft University of Technology
%
% Licensed under the Apache License, Version 2.0 (the "License");
% you may not use this file except in compliance with the License.
% You may obtain a copy of the License at
%
%      http://www.apache.org/licenses/LICENSE-2.0
%
% Unless required by applicable law or agreed to in writing, software
% distributed under the License is distributed on an "AS IS" BASIS,
% WITHOUT WARRANTIES OR CONDITIONS OF ANY KIND, either express or implied.
% See the License for the specific language governing permissions and
% limitations under the License.

function [v_a_dot, M_OB, v_k_W, pos_O,pos_W, v_k_B, chi_k, gamma_k,eta_EULER, ...
    v_k_O, chi_a_dot,gamma_a_dot,long_dot,lat_dot,h_tau_dot] = pmEOM(Va, alpha, ...
    beta, v_w_O, mu_a, F_a_B, F_p_B, F_t_W, chi_a, gamma_a, long, lat,h_tau, DE2019, ENVMT)
%pmEOM - Solve adapted equations of motion for a point mass dynamic system
%
% Inputs:
%    Va       - Aircraft velocity component on body x axis
%    alpha    - Aircraft angle of attack
%    beta     - Aircraft side slip angle
%    v_w_O    - Wind velocity at aircraft in inertial reference frame
%    mu_a     - Roll angle aircraft in body reference frame
%    F_a_B    - Aerodynamic forces in body reference frame
%    F_p_B    - Propulsion forces in body reference frame
%    F_t_W    - Tether tension at aircraft in wind reference frame
%    chi_a    - Aerodynamic course heading
%    gamma_a  - Aerodynamic path angle
%    long     - Longtitude, ground station center of earth
%    lat      - Latitude, ground station center of earth
%    h_tau    - Distance from gound station
%    DE2019   - Aircraft parameters in data structure format
%    ENVMT    - Environmental properties
%
% Outputs:
%    v_a_dot        - Aircraft acceleration on body x axis
%    M_OB           - Transformation matrix between inertial and body
%                     reference frames
%    v_k_W          - Kinetic velocity in wind reference frame
%    pos_O          - Aircraft position in inertial reference frame
%    pos_W          - Aircraft position in wind reference frame
%    v_k_B          - Kinetic velocity in body reference frame
%    chi_k          - Kinetic course heading
%    gamma_k        - Kinetic path angle
%    eta_EULER      - Euler angles aircraft
%    v_k_O          - Kinetic velocity in inertial reference frame
%    chi_a_dot      - Time derivative course heading
%    gamma_a_dot    - Time derivative path angle
%    long_dot       - Time derivative longtitude
%    lat_dot        - Time derivative longtitude
%    h_tau_dot      - Time derivative distance from ground station
%
% Example: 
%    [v_a_dot, M_OB, v_k_W, pos_O,pos_W, v_k_B, chi_k, gamma_k,eta_EULER, ...
%     v_k_O, chi_a_dot,gamma_a_dot,long_dot,lat_dot,h_tau_dot] = pmEOM(Va, alpha, ...
%     beta, v_w_O, mu_a, F_a_B, F_p_B, F_t_W, chi_a, gamma_a, long, lat,h_tau, DE2019, ENVMT)
%
% Other m-files required: none
% Subfunctions: none
% MAT-files required: none
%
% Author: Sebastian Rapp, Phd.
% Delft University of Technology
% email address: s.rapp@tudelft.nl  

%------------- BEGIN CODE --------------

%% Pre-allocation of variables for codegen
beta_k= 0;
alpha_k= 0;
chi_k = 0;
gamma_k  = 0;
M_OB = zeros(3); 
eta_EULER = zeros(3,1); 

%% Initiate variables and transformation matrices
M_BA = [cos(alpha), 0, -sin(alpha); 
    0, 1, 0; 
 sin(alpha), -sin(alpha), cos(alpha)];

M_AB = M_BA.';

s_lat = sin(lat); 
s_long = sin(long); 
c_lat = cos(lat); 
c_long = cos(long); 

M_tauW = [-s_lat *c_long, -s_lat *s_long, c_lat;
    -s_long, c_long, 0;
    -c_lat*c_long, -c_lat*s_long, -s_lat ];

xi = ENVMT.windDirection_rad;
M_OW = [cos(xi), sin(xi), 0; 
    sin(xi), -cos(xi), 0; 
    0, 0, -1];
M_WO = M_OW; 

cos_ca = cos(chi_a); 
cos_ga = cos(gamma_a); 
sin_ca = sin(chi_a); 
sin_ga = sin(gamma_a); 

M_AbarO = [cos_ca*cos_ga, sin_ca*cos_ga, -sin_ga; 
    -sin_ca, cos_ca, 0; 
    cos_ca*sin_ga, sin_ca*sin_ga, cos_ga];
M_OAbar = M_AbarO';
M_AbarA = [1,0,0; 
            0, cos(mu_a), -sin(mu_a); 
            0, sin(mu_a), cos(mu_a)];
M_AAbar = M_AbarA';

%%
v_a_O = M_OAbar*[Va;0;0]; 
v_a_B = M_BA*[Va;0;0]; 
v_w_B = M_BA*M_AAbar*M_AbarO*v_w_O;
v_k_B = v_a_B + v_w_B; 
v_k_O = v_a_O + v_w_O; 
v_k_W = M_WO*v_k_O; 
Vk = norm(v_k_B); 

chi_k = atan2( v_k_O(2), v_k_O(1) ); 
gamma_k = -asin( 1/Vk*v_k_O(3) ); 


Ft_Abar = M_AbarO*M_OW*F_t_W;
Fa_Abar = M_AbarA*M_AB*F_a_B; 
Fp_Abar = M_AbarA*M_AB*F_p_B; 
Fg_Abar = M_AbarO*[0;0;DE2019.mass*ENVMT.g];

Ftot_Abar = Ft_Abar + Fg_Abar + Fa_Abar + Fp_Abar; 
x_dot_Abar = 1/DE2019.mass*diag([1,1/(Va*cos_ga),-1/Va]) * Ftot_Abar; 
% states are: Va, chi_a, gamma_a
v_a_dot = x_dot_Abar(1); 
chi_a_dot = x_dot_Abar(2);
gamma_a_dot = x_dot_Abar(3); 

v_k_tau =M_tauW*v_k_W;

long_dot = v_k_tau(2)/( abs(h_tau)*cos(lat));
lat_dot = v_k_tau(1)/abs(h_tau);
h_tau_dot = -v_k_tau(3);

pos_W= [cos(long)*cos(lat); sin(long)*cos(lat); sin(lat)]*h_tau;
pos_O = M_OW*pos_W; 
M_OB = M_OAbar * M_AbarA * M_AB;

%% Calculate euler angles, roll pitch yaw in inertial reference frame
PHI =  atan2( M_OB(3,2), M_OB(3,3) ); 
THETA = -asin( M_OB(3,1) ); 
PSI = atan2( M_OB(2,1), M_OB(1,1) ); 

eta_EULER = [PHI; THETA; PSI];

%------------- END CODE --------------
end
